simulink model "edge_detect_wrapper"  (R2025b)
settings: Solver=FixedStepDiscrete  StartTime=0.0  StopTime=1  RelTol=1e-3
undefined symbols (not defined in the file or in its folder): current_chunk, sobel_kx, sobel_ky
settings Model: Creator=adam  LastModifiedBy=adam

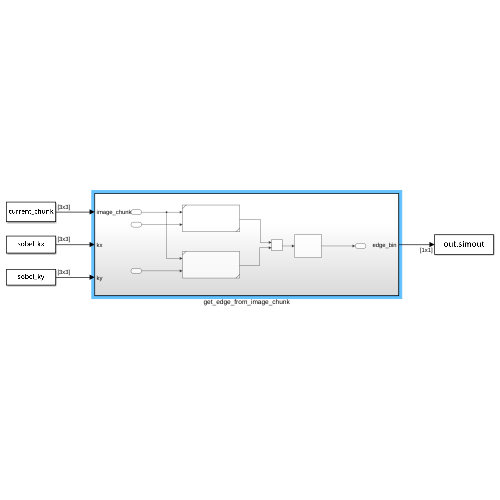
[thumbnail: Simulink's stored preview of the top-level diagram]
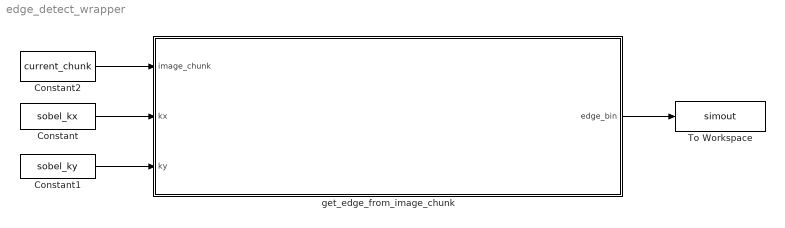
== system edge_detect_wrapper ==
  Constant : Constant  Value=sobel_kx  SampleTime=-1
  Constant1 : Constant  Value=sobel_ky  SampleTime=-1
  Constant2 : Constant  Value=current_chunk  SampleTime=-1
  To Workspace : ToWorkspace  VariableName=simout  SaveFormat=Timeseries  SampleTime=1
  get_edge_from_image_chunk : Subsystem
  wires:
  Constant2/1 -> get_edge_from_image_chunk/1(image_chunk)
  Constant/1 -> get_edge_from_image_chunk/2(kx)
  Constant1/1 -> get_edge_from_image_chunk/3(ky)
  get_edge_from_image_chunk/1(edge_bin) -> To Workspace/1

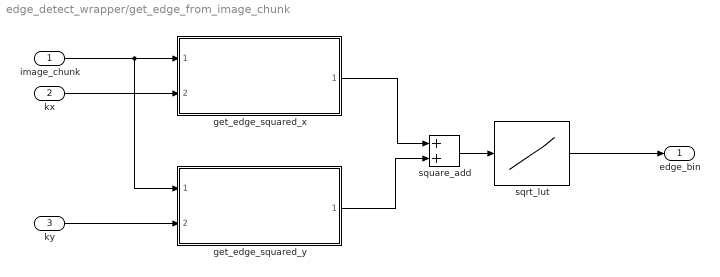
== system edge_detect_wrapper/get_edge_from_image_chunk ==
  image_chunk : Inport
  kx : Inport  Port=2
  ky : Inport  Port=3
  get_edge_squared_x : Subsystem  ReferencedSubsystem=get_edge_squared
  get_edge_squared_y : Subsystem  ReferencedSubsystem=get_edge_squared
  sqrt_lut : Lookup_n-D  NumberOfTableDimensions=1  BreakpointsForDimension1=[1:1024]  Table=sqrt([1:1024])  InternalRulePriority=Speed  RndMeth=Simplest
  square_add : Sum
  edge_bin : Outport
  wires:
  get_edge_squared_x/1 -> square_add/1
  square_add/1 -> sqrt_lut/1
  get_edge_squared_y/1 -> square_add/2
  sqrt_lut/1 -> edge_bin/1
  ky/1 -> get_edge_squared_y/2
  kx/1 -> get_edge_squared_x/2
  image_chunk/1 -> get_edge_squared_y/1, get_edge_squared_x/1
